simulink model "ex_2"  (R2019a)
settings: Solver=FixedStepAuto  StartTime=0.0  StopTime=20  FixedStep=1  RelTol=1e-3
settings Model: Creator=anton  LastModifiedBy=anton

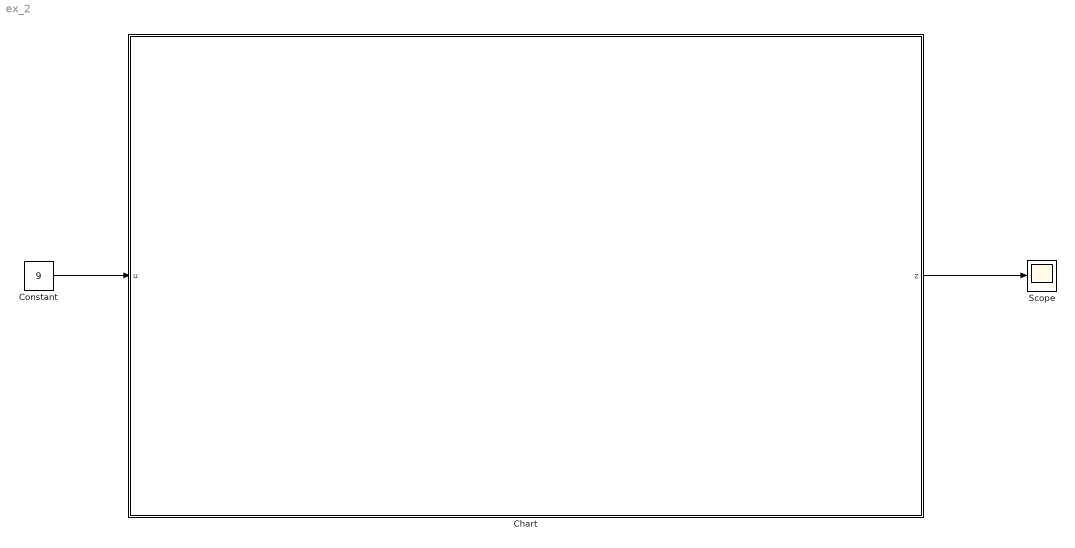
== system ex_2 ==
  Chart : Stateflow chart  BlockKeywords=__PRM__SERIALIZED__DATA__:Stateflow Chart,Stateflow Diagram  TreatAsAtomicUnit=on
  Constant : Constant  Value=9
  Scope : Scope
  wires:
  Constant/1 -> Chart/1(u)
  Chart/1(z) -> Scope/1

== stateflow chart ex_2/Chart ==
  state Init
    entry:
    n2 = rem(n,2);
    y=false;
    exit:
    y=isequal(n,1);
  state Odd
    entry,during:
    n=3*(n-y)+1;
    n2=rem(n,2);
    z=n;
  state Even
    entry,during:
    n=n/2;
    n2=rem(n,2);
    z=n;
  (default) -> Init : {n=u;}
  Init -> (junction 6) [order 2]
  Init -> (junction 5) [order 1] : [n2==0]
  (junction 6) -> Odd
  (junction 5) -> Even
  Odd -> Even : [n2==0]
  Even -> Odd : [n2~=0]{y=isequal(n,1);}
  data: u input; n2 local; y local; n local; z output
